simulink library "sm_dump_trailer_lib"  (R2021b)
settings: Solver=VariableStepAuto  StartTime=0.0  StopTime=10.0  RelTol=1e-3  EnableMultiTasking=on
undefined symbols (not defined in the file or in its folder): X, Y, Z
libraries: sm_lib x25
settings Model: Creator=The MathWorks, Inc.  LastModifiedBy=The MathWorks, Inc.
settings SolverCC: AlgebraicLoopSolver=TrustRegion
settings DataIOCC: ReturnWorkspaceOutputs=off
settings DebuggingCC: SFMachineParentedDataDiag=warning  ArithmeticOperatorsInVariantConditions=warning
settings SFSimCC: SimUseLocalCustomCode=off  CustomCodeUndefinedFunction=UseInterfaceOnly
settings RTWCC: RTWUseLocalCustomCode=off
settings CodeAppCC: StateflowObjectComments=on
settings GRTTargetCC: TargetLangStandard=C89/C90 (ANSI)
settings ConfigComp: CovMetricSettings=dsw  CovSaveCumulativeToWorkspaceVar=on  CovSaveSingleToWorkspaceVar=on  CovExternalEMLEnable=off

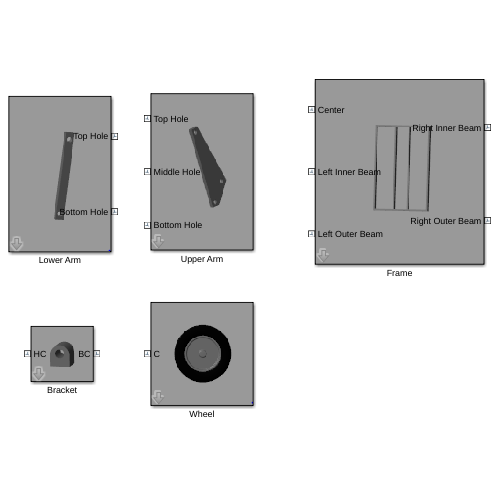
[thumbnail: Simulink's stored preview of the top-level diagram]
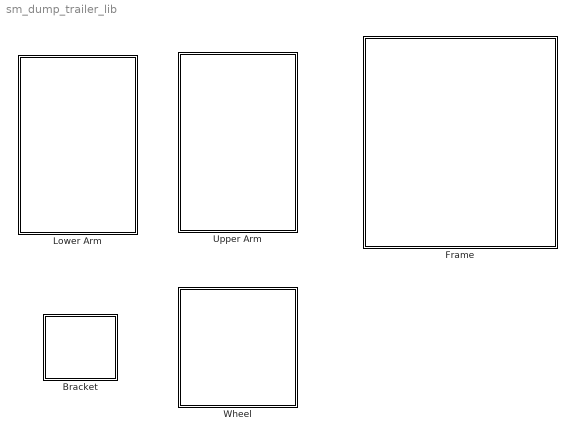
== system sm_dump_trailer_lib ==
  Bracket : Subsystem  mask(Bracket){Hbracket=0.05, Wbracket=0.045, Tbracket=0.045, Hhole=0.03, Rhole=0.01, rho=2700, bracketColor=[0.5 0.5 0.5]}
      mask prompts: Hbracket "Hbracket (m)"; Wbracket "Wbracket (m)"; Tbracket "Tbracket (m)"; Hhole "Hhole (m)"; Rhole "Rhole (m)"; rho "Density (kg/m^3)"; bracketColor "Bracket Color"
      mask help:
      | This block models a bracket.
      |
      | Attachment points are:
      | 1) The central point of the base (BC).
      | 2) The center point of the hole, which is configured for Revolute joints (HC).
      |
      | Click on Help to view a schematic of the bracket, its configurable dimension parameters and attachment points (in red).
      mask init:
      | points = 40;
      | 
      | y = Hbracket - (Wbracket/2);
      | 
      | outerVertices = [0 0;...
      |     Wbracket/2 0;...
      |     Wbracket/2 y;...
      |     Wbracket/2 Hbracket;...
      |     -Wbracket/2 Hbracket;...
      |     -Wbracket/2 y;...
      |     -Wbracket/2 0;...
      |     0 0];
      | 
      | outer = simmechanics.demohelpers.round_corners(outerVertices,[4 5],Wbracket/2,points);
      | 
      | thetaHole = linspace(1.5*pi,-0.5*pi,points);
      | 
      | hole = [Rhole*cos(thetaHole);...
      |     Rhole*sin(thetaHole)+Hhole]';
      | 
      | bracketPoints = [hole;outer];
      mask Help: web(fullfile(matlabroot,'toolbox','physmod','sm','smdemos','dump_trailer','demohelp','sm_dump_trailer_bracket.html'));
      mask DialogControl Tab01 Prompt: Dimensions
      mask DialogControl Tab02 Prompt: Material Properties
      mask Display:
      | image(fullfile(matlabroot,'toolbox','physmod','sm','smdemos','dump_trailer','images','sm_dump_trailer_bracket.png'));
      | port_label('lconn',1,'BC');
      | port_label('rconn',1,'HC');
  Frame : Subsystem  mask{W=2, L=3, H=0.15, T=0.05, d_innerbeams=0.5, rho=2700, color=[0.5 0.5 0.5]}
      mask prompts: W "Width (m)"; L "Length (m)"; H "Height (m)"; T "Beam thickness (m)"; d_innerbeams "Distance between inner beams (m)"; rho "Density (kg/m^3)"; color "Color [R G B]"
      mask Display: image(fullfile(matlabroot,'toolbox','physmod','sm','smdemos','dump_trailer','images','sm_dump_trailer_frame.png'));
  Lower Arm : Subsystem  mask{L=1, H=0.1, T=0.05, d_h2h=0.85, r_h=0.03, rho=8050, color=[0.5 0.5 0.5]}
      mask prompts: L "Length (m)"; H "Height (m)"; T "Thickness (m)"; d_h2h "Bottom hole to top hole distance (m)"; r_h "Hole radius (m)"; rho "Density (kg/m^3)"; color "Color [R G B]"
      mask init:
      | % points per hole
      | N = 40; 
      | 
      | % Cross-section
      | CS = [
      |     L/2, -H/2;...
      |     L/2, 0;...
      |     d_h2h/2 + r_h*cos(linspace(2*pi,0,N))', r_h*sin(linspace(2*pi,0,N))';...
      |     L/2, 0;...
      |     L/2, H/2;...
      |     -L/2, H/2;...
      |     -L/2, 0;...
      |     -d_h2h/2 + r_h*cos(linspace(pi,-pi,N))', r_h*sin(linspace(pi,-pi,N))';...
      |     -L/2, 0;...
      |     -L/2, -H/2];
      mask Display: image(fullfile(matlabroot,'toolbox','physmod','sm','smdemos','dump_trailer','images','sm_dump_trailer_lower_arm.png'));
  Upper Arm : Subsystem  mask{d_top2bot=1, th_bot2mid=45, th_top2mid=15, T=0.05, r_h=0.03, rho=8050, color=[0.5 0.5 0.5]}
      mask prompts: d_top2bot "Bottom hole to top hole distance (m)"; th_bot2mid "Bottom hole to middle hole angle (deg)"; th_top2mid "Top hole to middle hole angle (deg)"; T "Thickness (m)"; r_h "Hole radius (m)"; rho "Density (kg/m^3)"; color "Color [R G B]"
      mask init:
      | % Points per hole
      | N = 41; 
      | 
      | % Distance from top hole to middle hole
      | d_top2mid = d_top2bot*sind(th_bot2mid)/(sind(180-th_bot2mid-th_top2mid));
      | 
      | % Hole centers for cross-section
      | c_top = [0,0]; % top
      | c_bot = [d_top2bot, 0];
      | c_mid = [d_top2mid*cosd(th_top2mid), d_top2mid*sind(th_top2mid)];
      | 
      | % Vertices for holes
      | phi_top = linspace(180,-180,N)';
      | v_top = c_top + r_h*[cosd(phi_top), sind(phi_top)];
      | phi_mid = linspace(90,-270,N)';
      | v_mid = c_mid + r_h*[cosd(phi_mid), sind(phi_mid)];
      | phi_bot = linspace(360,0,N)';
      | v_bot = c_bot + r_h*[cosd(phi_bot), sind(phi_bot)];
      | 
      | % Vertices for cross section (counter-clockwise starting in front top
      | % corner)
      | CS = [...
      |     c_top + [-2*r_h, -2*r_h]; % front top corner
      |     c_bot + [2*r_h, -2*r_h]; % front bottom corner
      |     c_bot + [2*r_h,0]; % midpoint bottom
      |     v_bot; % bottom hole
      |     c_bot + [2*r_h,0]; % midpoint bottom
      |     c_bot + [2*r_h,2*r_h]; % back bottom corner
      |     c_mid + [3*r_h*sind((th_bot2mid-th_top2mid)/2),3*r_h*cosd((th_bot2mid-th_top2mid)/2)]; % back middle corner
      |     v_mid; % middle hole
      |     c_mid + [3*r_h*sind((th_bot2mid-th_top2mid)/2),3*r_h*cosd((th_bot2mid-th_top2mid)/2)]; % back middle corner
      |     c_top + [-2*r_h, 2*r_h]; %back top corner
      |     c_top + [-2*r_h,0]; % midpoint top
      |     v_top; % top hole
      |     c_top + [-2*r_h,0]; % midpoint top
      | ];
      mask Display: image(fullfile(matlabroot,'toolbox','physmod','sm','smdemos','dump_trailer','images','sm_dump_trailer_upper_arm.png'));
  Wheel : Subsystem  mask{r_i=0.25, r_o=0.4, w=0.15, r_c=0.01, rho_tire=1000, color_tire=[0 0 0], rho_hub=2700, color_hub=[0.5 0.5 0.5]}
      mask prompts: r_i "Inner radius (m)"; r_o "Outer radius (m)"; w "Width (m)"; r_c "Chamfer/fillet radius (m)"; rho_tire "Density (kg/m^3)"; color_tire "Color [R G B]"; rho_hub "Density (kg/m^3)"; color_hub "Color [R G B]"
      mask init:
      | % Tire cross-section
      | CS_tire = [...
      |     r_i,-w/2;
      |     r_o,-w/2;
      |     r_o,w/2;
      |     r_i,w/2];
      | CS_tire = simmechanics.demohelpers.round_corners(CS_tire,1:4,r_c,10);
      | 
      | % Hub cross-section
      | CS_hub = [...
      |     0,-w/3;
      |     1/5*r_i,-w/3;
      |     1/5*r_i,-w/8;
      |     1/2*r_i,-w/8;
      |     1/2*r_i,-w/6;
      |     9/10*r_i,-w/6;
      |     9/10*r_i,-w/2+r_c;
      |     r_i,-w/2+r_c;
      |     r_i,w/2-r_c;
      |     9/10*r_i,w/2-r_c;
      |     9/10*r_i,w/6;
      |     1/2*r_i,w/6;
      |     1/2*r_i,w/8;
      |     1/5*r_i,w/8;
      |     1/5*r_i,w/3;
      |     0,w/3];
      | CS_hub = simmechanics.demohelpers.round_corners(CS_hub,[2,3,6,7,10,11,14,15],r_c,10);
      mask DialogControl Container4 Prompt: Tire
      mask DialogControl Container7 Prompt: Hub
      mask Display: image(fullfile(matlabroot,'toolbox','physmod','sm','smdemos','dump_trailer','images','sm_dump_trailer_wheel.png'));

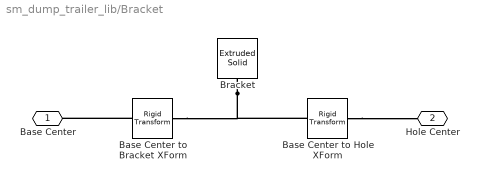
== system sm_dump_trailer_lib/Bracket ==
  Base Center to Bracket XForm : sm_lib/Frames and Transforms/Rigid Transform  TranslationMethod=None  TranslationStandardOffset=0  TranslationLengthUnit=m  TranslationStandardAxis=-Y  TranslationCartesianOffset=[0 0 0]  TranslationROffset=0  TranslationROffsetUnits=m  TranslationZOffset=0  TranslationZOffsetUnits=m  TranslationThetaOffset=0  TranslationThetaOffsetUnits=deg  RotationMethod=AlignedAxes  RotationAngleUnits=deg  RotationStandardAxis=+X  RotationAngle=90  RotationArbitraryAxis=[0 0 1]  FollAlignAxisA=+X  BaseAlignAxisA=+X  FollAlignAxisB=+Y  BaseAlignAxisB=+Z  RotationSequenceAxes=FollowerAxes  RotationSequence=XYX  RotationSequenceAngles=[0 0 0]  RotationSequenceAnglesUnits=deg  RotationMatrix=[1 0 0; 0 1 0; 0 0 1]
  Base Center to Hole XForm : sm_lib/Frames and Transforms/Rigid Transform  TranslationMethod=StandardAxis  TranslationStandardOffset=Hhole  TranslationLengthUnit=m  TranslationStandardAxis=+Y  TranslationCartesianOffset=[0 0 0]  TranslationROffset=0  TranslationROffsetUnits=m  TranslationZOffset=0  TranslationZOffsetUnits=m  TranslationThetaOffset=0  TranslationThetaOffsetUnits=deg  RotationMethod=None  RotationAngleUnits=deg  RotationStandardAxis=+X  RotationAngle=90  RotationArbitraryAxis=[0 0 1]  FollAlignAxisA=+X  BaseAlignAxisA=+X  FollAlignAxisB=+Y  BaseAlignAxisB=+Z  RotationSequenceAxes=FollowerAxes  RotationSequence=XYX  RotationSequenceAngles=[0 0 0]  RotationSequenceAnglesUnits=deg  RotationMatrix=[1 0 0; 0 1 0; 0 0 1]
  Bracket : sm_lib/Body Elements/Extruded Solid  GraphicAmbientColor=[0.15 0.15 0.15 1.0]  BasedOnType=Density  CenterOfMass=[0 0 0]  CenterOfMassUnits=m  GraphicDiffuseColor=bracketColor  ExportConvexHullGeometry=off  ExtrusionCrossSection=bracketPoints  ExtrusionCrossSectionUnits=m  Density=rho  DensityUnits=kg/(m^3)  DoExposeReferenceFrame=on  GraphicEmissiveColor=[0.0 0.0 0.0 1.0]  ExportEntireGeometry=off  ExtrusionLength=Tbracket  ExtrusionLengthUnits=m  ExtrusionType=General  SerializedFrames=<Frames/>  MarkerShape=Sphere  MarkerSize=10  GraphicType=FromGeometry  InertiaType=CalculateFromGeometry  Mass=1  MassUnits=kg  MomentsOfInertia=[1 1 1]  MomentsOfInertiaUnits=kg*m^2  PolygonNumSides=3  GraphicOpacity=1.0  PolygonOuterRadius=1  PolygonOuterRadiusUnits=m  ProductsOfInertia=[0 0 0]  ProductsOfInertiaUnits=kg*m^2  GraphicShininess=75  GraphicSpecularColor=[0.5 0.5 0.5 1.0]  GraphicVisPropType=SimpleVisualProperties
  Base Center : PMIOPort  Side=Left
  Hole Center : PMIOPort  Port=2  Side=Right
  connections:
  Base Center to Bracket XForm/LConn1 -- Base Center/RConn1
  Base Center to Hole XForm/RConn1 -- Hole Center/RConn1
  Bracket/RConn1 -- Base Center to Bracket XForm/RConn1 -- Base Center to Hole XForm/LConn1

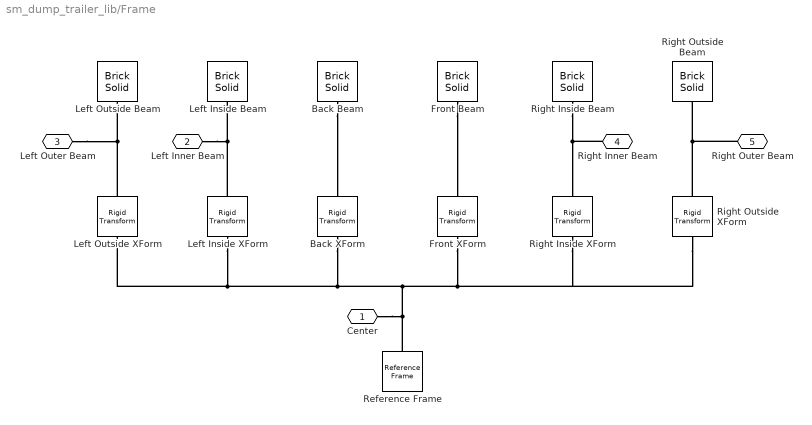
== system sm_dump_trailer_lib/Frame ==
  Back Beam : sm_lib/Body Elements/Brick Solid  GraphicAmbientColor=[0.15 0.15 0.15 1.0]  BasedOnType=Density  BrickDimensions=[W T H]  BrickDimensionUnits=m  CenterOfMass=[0 0 0]  CenterOfMassUnits=m  GraphicDiffuseColor=color  Density=rho  DensityUnits=kg/m^3  DoExposeReferenceFrame=on  GraphicEmissiveColor=[0.0 0.0 0.0 1.0]  ExportEntireGeometry=off  SerializedFrames=<Frames/>  MarkerShape=Sphere  MarkerSize=10  GraphicType=FromGeometry  InertiaType=CalculateFromGeometry  Mass=1  MassUnits=kg  MomentsOfInertia=[1 1 1]  MomentsOfInertiaUnits=kg*m^2  GraphicOpacity=1.0  ProductsOfInertia=[1 1 1]  ProductsOfInertiaUnits=kg*m^2  GraphicShininess=75  GraphicSpecularColor=[0.5 0.5 0.5 1.0]  GraphicVisPropType=SimpleVisualProperties
  Back XForm : sm_lib/Frames and Transforms/Rigid Transform  TranslationMethod=Cartesian  TranslationStandardOffset=0  TranslationLengthUnit=m  TranslationStandardAxis=+Z  TranslationCartesianOffset=[0 (L-T)/2 0]  TranslationROffset=0  TranslationROffsetUnits=m  TranslationZOffset=0  TranslationZOffsetUnits=m  TranslationThetaOffset=0  TranslationThetaOffsetUnits=deg  RotationMethod=None  RotationAngleUnits=deg  RotationStandardAxis=+Z  RotationAngle=0.0  RotationArbitraryAxis=[0 0 1]  FollAlignAxisA=+X  BaseAlignAxisA=+Y  FollAlignAxisB=+Y  BaseAlignAxisB=+Z  RotationSequenceAxes=FollowerAxes  RotationSequence=XYX  RotationSequenceAngles=[0 0 0]  RotationSequenceAnglesUnits=deg  RotationMatrix=[1 0 0; 0 1 0; 0 0 1]
  Front Beam : sm_lib/Body Elements/Brick Solid  GraphicAmbientColor=[0.15 0.15 0.15 1.0]  BasedOnType=Density  BrickDimensions=[W T H]  BrickDimensionUnits=m  CenterOfMass=[0 0 0]  CenterOfMassUnits=m  GraphicDiffuseColor=color  Density=rho  DensityUnits=kg/m^3  DoExposeReferenceFrame=on  GraphicEmissiveColor=[0.0 0.0 0.0 1.0]  ExportEntireGeometry=off  SerializedFrames=<Frames/>  MarkerShape=Sphere  MarkerSize=10  GraphicType=FromGeometry  InertiaType=CalculateFromGeometry  Mass=1  MassUnits=kg  MomentsOfInertia=[1 1 1]  MomentsOfInertiaUnits=kg*m^2  GraphicOpacity=1.0  ProductsOfInertia=[1 1 1]  ProductsOfInertiaUnits=kg*m^2  GraphicShininess=75  GraphicSpecularColor=[0.5 0.5 0.5 1.0]  GraphicVisPropType=SimpleVisualProperties
  Front XForm : sm_lib/Frames and Transforms/Rigid Transform  TranslationMethod=Cartesian  TranslationStandardOffset=0  TranslationLengthUnit=m  TranslationStandardAxis=+Z  TranslationCartesianOffset=[0 -(L-T)/2 0]  TranslationROffset=0  TranslationROffsetUnits=m  TranslationZOffset=0  TranslationZOffsetUnits=m  TranslationThetaOffset=0  TranslationThetaOffsetUnits=deg  RotationMethod=None  RotationAngleUnits=deg  RotationStandardAxis=+Z  RotationAngle=0.0  RotationArbitraryAxis=[0 0 1]  FollAlignAxisA=+X  BaseAlignAxisA=+Y  FollAlignAxisB=+Y  BaseAlignAxisB=+Z  RotationSequenceAxes=FollowerAxes  RotationSequence=XYX  RotationSequenceAngles=[0 0 0]  RotationSequenceAnglesUnits=deg  RotationMatrix=[1 0 0; 0 1 0; 0 0 1]
  Left Inside Beam : sm_lib/Body Elements/Brick Solid  GraphicAmbientColor=[0.15 0.15 0.15 1.0]  BasedOnType=Density  BrickDimensions=[L-2*T T H]  BrickDimensionUnits=m  CenterOfMass=[0 0 0]  CenterOfMassUnits=m  GraphicDiffuseColor=color  Density=rho  DensityUnits=kg/m^3  DoExposeReferenceFrame=on  GraphicEmissiveColor=[0.0 0.0 0.0 1.0]  ExportEntireGeometry=off  SerializedFrames=<Frames/>  MarkerShape=Sphere  MarkerSize=10  GraphicType=FromGeometry  InertiaType=CalculateFromGeometry  Mass=1  MassUnits=kg  MomentsOfInertia=[1 1 1]  MomentsOfInertiaUnits=kg*m^2  GraphicOpacity=1.0  ProductsOfInertia=[1 1 1]  ProductsOfInertiaUnits=kg*m^2  GraphicShininess=75  GraphicSpecularColor=[0.5 0.5 0.5 1.0]  GraphicVisPropType=SimpleVisualProperties
  Left Inside XForm : sm_lib/Frames and Transforms/Rigid Transform  TranslationMethod=Cartesian  TranslationStandardOffset=0  TranslationLengthUnit=m  TranslationStandardAxis=+Z  TranslationCartesianOffset=[-d_innerbeams/2 0 0]  TranslationROffset=0  TranslationROffsetUnits=m  TranslationZOffset=0  TranslationZOffsetUnits=m  TranslationThetaOffset=0  TranslationThetaOffsetUnits=deg  RotationMethod=StandardAxis  RotationAngleUnits=deg  RotationStandardAxis=+Z  RotationAngle=90  RotationArbitraryAxis=[0 0 1]  FollAlignAxisA=+X  BaseAlignAxisA=+Y  FollAlignAxisB=+Y  BaseAlignAxisB=+Z  RotationSequenceAxes=FollowerAxes  RotationSequence=XYX  RotationSequenceAngles=[0 0 0]  RotationSequenceAnglesUnits=deg  RotationMatrix=[1 0 0; 0 1 0; 0 0 1]
  Left Outside Beam : sm_lib/Body Elements/Brick Solid  GraphicAmbientColor=[0.15 0.15 0.15 1.0]  BasedOnType=Density  BrickDimensions=[L-2*T T H]  BrickDimensionUnits=m  CenterOfMass=[0 0 0]  CenterOfMassUnits=m  GraphicDiffuseColor=color  Density=rho  DensityUnits=kg/m^3  DoExposeReferenceFrame=on  GraphicEmissiveColor=[0.0 0.0 0.0 1.0]  ExportEntireGeometry=off  SerializedFrames=<Frames/>  MarkerShape=Sphere  MarkerSize=10  GraphicType=FromGeometry  InertiaType=CalculateFromGeometry  Mass=1  MassUnits=kg  MomentsOfInertia=[1 1 1]  MomentsOfInertiaUnits=kg*m^2  GraphicOpacity=1.0  ProductsOfInertia=[1 1 1]  ProductsOfInertiaUnits=kg*m^2  GraphicShininess=75  GraphicSpecularColor=[0.5 0.5 0.5 1.0]  GraphicVisPropType=SimpleVisualProperties
  Left Outside XForm : sm_lib/Frames and Transforms/Rigid Transform  TranslationMethod=Cartesian  TranslationStandardOffset=0  TranslationLengthUnit=m  TranslationStandardAxis=+Z  TranslationCartesianOffset=[-(W-T)/2 0 0]  TranslationROffset=0  TranslationROffsetUnits=m  TranslationZOffset=0  TranslationZOffsetUnits=m  TranslationThetaOffset=0  TranslationThetaOffsetUnits=deg  RotationMethod=StandardAxis  RotationAngleUnits=deg  RotationStandardAxis=+Z  RotationAngle=90  RotationArbitraryAxis=[0 0 1]  FollAlignAxisA=+X  BaseAlignAxisA=+Y  FollAlignAxisB=+Y  BaseAlignAxisB=+Z  RotationSequenceAxes=FollowerAxes  RotationSequence=XYX  RotationSequenceAngles=[0 0 0]  RotationSequenceAnglesUnits=deg  RotationMatrix=[1 0 0; 0 1 0; 0 0 1]
  Reference Frame : sm_lib/Frames and Transforms/Reference Frame
  Right Inside Beam : sm_lib/Body Elements/Brick Solid  GraphicAmbientColor=[0.15 0.15 0.15 1.0]  BasedOnType=Density  BrickDimensions=[L-2*T T H]  BrickDimensionUnits=m  CenterOfMass=[0 0 0]  CenterOfMassUnits=m  GraphicDiffuseColor=color  Density=rho  DensityUnits=kg/m^3  DoExposeReferenceFrame=on  GraphicEmissiveColor=[0.0 0.0 0.0 1.0]  ExportEntireGeometry=off  SerializedFrames=<Frames/>  MarkerShape=Sphere  MarkerSize=10  GraphicType=FromGeometry  InertiaType=CalculateFromGeometry  Mass=1  MassUnits=kg  MomentsOfInertia=[1 1 1]  MomentsOfInertiaUnits=kg*m^2  GraphicOpacity=1.0  ProductsOfInertia=[1 1 1]  ProductsOfInertiaUnits=kg*m^2  GraphicShininess=75  GraphicSpecularColor=[0.5 0.5 0.5 1.0]  GraphicVisPropType=SimpleVisualProperties
  Right Inside XForm : sm_lib/Frames and Transforms/Rigid Transform  TranslationMethod=Cartesian  TranslationStandardOffset=0  TranslationLengthUnit=m  TranslationStandardAxis=+Z  TranslationCartesianOffset=[d_innerbeams/2 0 0]  TranslationROffset=0  TranslationROffsetUnits=m  TranslationZOffset=0  TranslationZOffsetUnits=m  TranslationThetaOffset=0  TranslationThetaOffsetUnits=deg  RotationMethod=StandardAxis  RotationAngleUnits=deg  RotationStandardAxis=+Z  RotationAngle=90  RotationArbitraryAxis=[0 0 1]  FollAlignAxisA=+X  BaseAlignAxisA=+Y  FollAlignAxisB=+Y  BaseAlignAxisB=+Z  RotationSequenceAxes=FollowerAxes  RotationSequence=XYX  RotationSequenceAngles=[0 0 0]  RotationSequenceAnglesUnits=deg  RotationMatrix=[1 0 0; 0 1 0; 0 0 1]
  Right Outside Beam : sm_lib/Body Elements/Brick Solid  GraphicAmbientColor=[0.15 0.15 0.15 1.0]  BasedOnType=Density  BrickDimensions=[L-2*T T H]  BrickDimensionUnits=m  CenterOfMass=[0 0 0]  CenterOfMassUnits=m  GraphicDiffuseColor=color  Density=rho  DensityUnits=kg/m^3  DoExposeReferenceFrame=on  GraphicEmissiveColor=[0.0 0.0 0.0 1.0]  ExportEntireGeometry=off  SerializedFrames=<Frames/>  MarkerShape=Sphere  MarkerSize=10  GraphicType=FromGeometry  InertiaType=CalculateFromGeometry  Mass=1  MassUnits=kg  MomentsOfInertia=[1 1 1]  MomentsOfInertiaUnits=kg*m^2  GraphicOpacity=1.0  ProductsOfInertia=[1 1 1]  ProductsOfInertiaUnits=kg*m^2  GraphicShininess=75  GraphicSpecularColor=[0.5 0.5 0.5 1.0]  GraphicVisPropType=SimpleVisualProperties
  Right Outside XForm : sm_lib/Frames and Transforms/Rigid Transform  TranslationMethod=Cartesian  TranslationStandardOffset=0  TranslationLengthUnit=m  TranslationStandardAxis=+Z  TranslationCartesianOffset=[(W-T)/2 0 0]  TranslationROffset=0  TranslationROffsetUnits=m  TranslationZOffset=0  TranslationZOffsetUnits=m  TranslationThetaOffset=0  TranslationThetaOffsetUnits=deg  RotationMethod=StandardAxis  RotationAngleUnits=deg  RotationStandardAxis=+Z  RotationAngle=90  RotationArbitraryAxis=[0 0 1]  FollAlignAxisA=+X  BaseAlignAxisA=+Y  FollAlignAxisB=+Y  BaseAlignAxisB=+Z  RotationSequenceAxes=FollowerAxes  RotationSequence=XYX  RotationSequenceAngles=[0 0 0]  RotationSequenceAnglesUnits=deg  RotationMatrix=[1 0 0; 0 1 0; 0 0 1]
  Center : PMIOPort  Side=Left
  Left Inner Beam : PMIOPort  Port=2  Side=Left
  Left Outer Beam : PMIOPort  Port=3  Side=Left
  Right Inner Beam : PMIOPort  Port=4  Side=Right
  Right Outer Beam : PMIOPort  Port=5  Side=Right
  connections:
  Left Outside XForm/RConn1 -- Left Outer Beam/RConn1 -- Left Outside Beam/RConn1
  Reference Frame/RConn1 -- Center/RConn1 -- Right Outside XForm/LConn1 -- Right Inside XForm/LConn1 -- Front XForm/LConn1 -- Back XForm/LConn1 -- Left Outside XForm/LConn1 -- Left Inside XForm/LConn1
  Left Inside XForm/RConn1 -- Left Inner Beam/RConn1 -- Left Inside Beam/RConn1
  Back Beam/RConn1 -- Back XForm/RConn1
  Front Beam/RConn1 -- Front XForm/RConn1
  Right Inside Beam/RConn1 -- Right Inner Beam/RConn1 -- Right Inside XForm/RConn1
  Right Outside XForm/RConn1 -- Right Outer Beam/RConn1 -- Right Outside Beam/RConn1

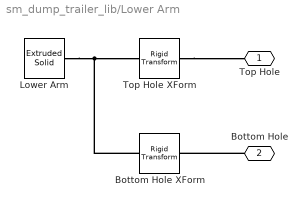
== system sm_dump_trailer_lib/Lower Arm ==
  Bottom Hole XForm : sm_lib/Frames and Transforms/Rigid Transform  TranslationMethod=StandardAxis  TranslationStandardOffset=d_h2h/2  TranslationLengthUnit=m  TranslationStandardAxis=-X  TranslationCartesianOffset=[0 0 0]  TranslationROffset=0  TranslationROffsetUnits=m  TranslationZOffset=0  TranslationZOffsetUnits=m  TranslationThetaOffset=0  TranslationThetaOffsetUnits=deg  RotationMethod=None  RotationAngleUnits=deg  RotationStandardAxis=+Z  RotationAngle=0.0  RotationArbitraryAxis=[0 0 1]  FollAlignAxisA=+X  BaseAlignAxisA=+Y  FollAlignAxisB=+Y  BaseAlignAxisB=+Z  RotationSequenceAxes=FollowerAxes  RotationSequence=XYX  RotationSequenceAngles=[0 0 0]  RotationSequenceAnglesUnits=deg  RotationMatrix=[1 0 0; 0 1 0; 0 0 1]
  Lower Arm : sm_lib/Body Elements/Extruded Solid  GraphicAmbientColor=[0.15 0.15 0.15 1.0]  BasedOnType=Density  CenterOfMass=[0 0 0]  CenterOfMassUnits=m  GraphicDiffuseColor=color  ExportConvexHullGeometry=off  ExtrusionCrossSection=CS  ExtrusionCrossSectionUnits=m  Density=rho  DensityUnits=kg/m^3  DoExposeReferenceFrame=on  GraphicEmissiveColor=[0.0 0.0 0.0 1.0]  ExportEntireGeometry=off  ExtrusionLength=T  ExtrusionLengthUnits=m  ExtrusionType=General  SerializedFrames=<Frames/>  MarkerShape=Sphere  MarkerSize=10  GraphicType=FromGeometry  InertiaType=CalculateFromGeometry  Mass=1  MassUnits=kg  MomentsOfInertia=[1 1 1]  MomentsOfInertiaUnits=kg*m^2  PolygonNumSides=3  GraphicOpacity=1.0  PolygonOuterRadius=1  PolygonOuterRadiusUnits=m  ProductsOfInertia=[1 1 1]  ProductsOfInertiaUnits=kg*m^2  GraphicShininess=75  GraphicSpecularColor=[0.5 0.5 0.5 1.0]  GraphicVisPropType=SimpleVisualProperties
  Top Hole XForm : sm_lib/Frames and Transforms/Rigid Transform  TranslationMethod=StandardAxis  TranslationStandardOffset=d_h2h/2  TranslationLengthUnit=m  TranslationStandardAxis=+X  TranslationCartesianOffset=[0 0 0]  TranslationROffset=0  TranslationROffsetUnits=m  TranslationZOffset=0  TranslationZOffsetUnits=m  TranslationThetaOffset=0  TranslationThetaOffsetUnits=deg  RotationMethod=None  RotationAngleUnits=deg  RotationStandardAxis=+Z  RotationAngle=0.0  RotationArbitraryAxis=[0 0 1]  FollAlignAxisA=+X  BaseAlignAxisA=+Y  FollAlignAxisB=+Y  BaseAlignAxisB=+Z  RotationSequenceAxes=FollowerAxes  RotationSequence=XYX  RotationSequenceAngles=[0 0 0]  RotationSequenceAnglesUnits=deg  RotationMatrix=[1 0 0; 0 1 0; 0 0 1]
  Top Hole : PMIOPort  Side=Right
  Bottom Hole : PMIOPort  Port=2  Side=Right
  connections:
  Top Hole XForm/RConn1 -- Top Hole/RConn1
  Bottom Hole/RConn1 -- Bottom Hole XForm/RConn1
  Lower Arm/RConn1 -- Bottom Hole XForm/LConn1 -- Top Hole XForm/LConn1

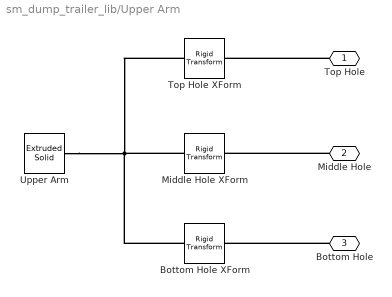
== system sm_dump_trailer_lib/Upper Arm ==
  Bottom Hole XForm : sm_lib/Frames and Transforms/Rigid Transform  TranslationMethod=Cartesian  TranslationStandardOffset=0  TranslationLengthUnit=m  TranslationStandardAxis=+Z  TranslationCartesianOffset=[c_bot,0]  TranslationROffset=0  TranslationROffsetUnits=m  TranslationZOffset=0  TranslationZOffsetUnits=m  TranslationThetaOffset=0  TranslationThetaOffsetUnits=deg  RotationMethod=None  RotationAngleUnits=deg  RotationStandardAxis=+Z  RotationAngle=0.0  RotationArbitraryAxis=[0 0 1]  FollAlignAxisA=+X  BaseAlignAxisA=+Y  FollAlignAxisB=+Y  BaseAlignAxisB=+Z  RotationSequenceAxes=FollowerAxes  RotationSequence=XYX  RotationSequenceAngles=[0 0 0]  RotationSequenceAnglesUnits=deg  RotationMatrix=[1 0 0; 0 1 0; 0 0 1]
  Middle Hole XForm : sm_lib/Frames and Transforms/Rigid Transform  TranslationMethod=Cartesian  TranslationStandardOffset=0  TranslationLengthUnit=m  TranslationStandardAxis=+Z  TranslationCartesianOffset=[c_mid,0]  TranslationROffset=0  TranslationROffsetUnits=m  TranslationZOffset=0  TranslationZOffsetUnits=m  TranslationThetaOffset=0  TranslationThetaOffsetUnits=deg  RotationMethod=None  RotationAngleUnits=deg  RotationStandardAxis=+Z  RotationAngle=0.0  RotationArbitraryAxis=[0 0 1]  FollAlignAxisA=+X  BaseAlignAxisA=+Y  FollAlignAxisB=+Y  BaseAlignAxisB=+Z  RotationSequenceAxes=FollowerAxes  RotationSequence=XYX  RotationSequenceAngles=[0 0 0]  RotationSequenceAnglesUnits=deg  RotationMatrix=[1 0 0; 0 1 0; 0 0 1]
  Top Hole XForm : sm_lib/Frames and Transforms/Rigid Transform  TranslationMethod=Cartesian  TranslationStandardOffset=0  TranslationLengthUnit=m  TranslationStandardAxis=+Z  TranslationCartesianOffset=[c_top,0]  TranslationROffset=0  TranslationROffsetUnits=m  TranslationZOffset=0  TranslationZOffsetUnits=m  TranslationThetaOffset=0  TranslationThetaOffsetUnits=deg  RotationMethod=None  RotationAngleUnits=deg  RotationStandardAxis=+Z  RotationAngle=0.0  RotationArbitraryAxis=[0 0 1]  FollAlignAxisA=+X  BaseAlignAxisA=+Y  FollAlignAxisB=+Y  BaseAlignAxisB=+Z  RotationSequenceAxes=FollowerAxes  RotationSequence=XYX  RotationSequenceAngles=[0 0 0]  RotationSequenceAnglesUnits=deg  RotationMatrix=[1 0 0; 0 1 0; 0 0 1]
  Upper Arm : sm_lib/Body Elements/Extruded Solid  GraphicAmbientColor=[0.15 0.15 0.15 1.0]  BasedOnType=Density  CenterOfMass=[0 0 0]  CenterOfMassUnits=m  GraphicDiffuseColor=color  ExportConvexHullGeometry=off  ExtrusionCrossSection=CS  ExtrusionCrossSectionUnits=m  Density=rho  DensityUnits=kg/m^3  DoExposeReferenceFrame=on  GraphicEmissiveColor=[0.0 0.0 0.0 1.0]  ExportEntireGeometry=off  ExtrusionLength=T  ExtrusionLengthUnits=m  ExtrusionType=General  SerializedFrames=<Frames/>  MarkerShape=Sphere  MarkerSize=10  GraphicType=FromGeometry  InertiaType=CalculateFromGeometry  Mass=1  MassUnits=kg  MomentsOfInertia=[1 1 1]  MomentsOfInertiaUnits=kg*m^2  PolygonNumSides=3  GraphicOpacity=1.0  PolygonOuterRadius=1  PolygonOuterRadiusUnits=m  ProductsOfInertia=[1 1 1]  ProductsOfInertiaUnits=kg*m^2  GraphicShininess=75  GraphicSpecularColor=[0.5 0.5 0.5 1.0]  GraphicVisPropType=SimpleVisualProperties
  Top Hole : PMIOPort  Side=Right
  Middle Hole : PMIOPort  Port=2  Side=Right
  Bottom Hole : PMIOPort  Port=3  Side=Right
  connections:
  Upper Arm/RConn1 -- Top Hole XForm/LConn1 -- Bottom Hole XForm/LConn1 -- Middle Hole XForm/LConn1
  Top Hole/RConn1 -- Top Hole XForm/RConn1
  Middle Hole/RConn1 -- Middle Hole XForm/RConn1
  Bottom Hole/RConn1 -- Bottom Hole XForm/RConn1

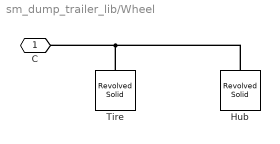
== system sm_dump_trailer_lib/Wheel ==
  Hub : sm_lib/Body Elements/Revolved Solid  GraphicAmbientColor=[0.15 0.15 0.15 1.0]  BasedOnType=Density  CenterOfMass=[0 0 0]  CenterOfMassUnits=m  GraphicDiffuseColor=color_hub  ExportConvexHullGeometry=off  Density=rho_hub  DensityUnits=kg/m^3  DoExposeReferenceFrame=on  GraphicEmissiveColor=[0.0 0.0 0.0 1.0]  ExportEntireGeometry=off  SerializedFrames=<Frames/>  MarkerShape=Sphere  MarkerSize=10  GraphicType=FromGeometry  InertiaType=CalculateFromGeometry  Mass=1  MassUnits=kg  MomentsOfInertia=[1 1 1]  MomentsOfInertiaUnits=kg*m^2  GraphicOpacity=1.0  ProductsOfInertia=[1 1 1]  ProductsOfInertiaUnits=kg*m^2  RevolutionCrossSection=CS_hub  RevolutionCrossSectionUnits=m  RevolutionAngle=180  RevolutionAngleUnits=deg  RevolutionExtent=Full  GraphicShininess=75  GraphicSpecularColor=[0.5 0.5 0.5 1.0]  GraphicVisPropType=SimpleVisualProperties
  Tire : sm_lib/Body Elements/Revolved Solid  GraphicAmbientColor=[0.15 0.15 0.15 1.0]  BasedOnType=Density  CenterOfMass=[0 0 0]  CenterOfMassUnits=m  GraphicDiffuseColor=color_tire  ExportConvexHullGeometry=off  Density=rho_tire  DensityUnits=kg/m^3  DoExposeReferenceFrame=on  GraphicEmissiveColor=[0.0 0.0 0.0 1.0]  ExportEntireGeometry=off  SerializedFrames=<Frames/>  MarkerShape=Sphere  MarkerSize=10  GraphicType=FromGeometry  InertiaType=CalculateFromGeometry  Mass=1  MassUnits=kg  MomentsOfInertia=[1 1 1]  MomentsOfInertiaUnits=kg*m^2  GraphicOpacity=1.0  ProductsOfInertia=[1 1 1]  ProductsOfInertiaUnits=kg*m^2  RevolutionCrossSection=CS_tire  RevolutionCrossSectionUnits=m  RevolutionAngle=180  RevolutionAngleUnits=deg  RevolutionExtent=Full  GraphicShininess=75  GraphicSpecularColor=[0.5 0.5 0.5 1.0]  GraphicVisPropType=SimpleVisualProperties
  C : PMIOPort  Side=Left
  connections:
  Tire/RConn1 -- C/RConn1 -- Hub/RConn1
